simulink model "qref_Model"  (R2024a)
settings: Solver=VariableStepAuto  StartTime=0.0  StopTime=10.0  RelTol=1e-3
libraries: sharedtransform x2, aerolibconvert2 x1
settings Model: Creator=hendr  LastModifiedBy=hendr

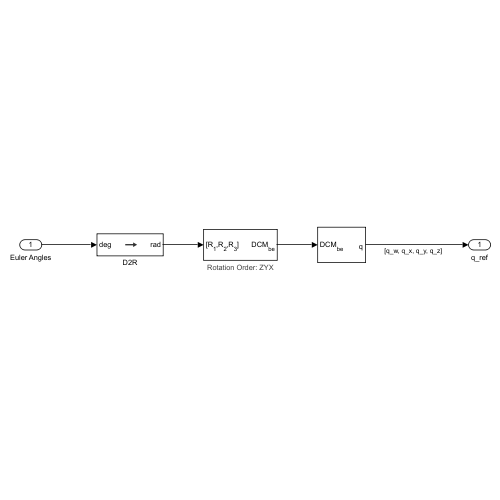
[thumbnail: Simulink's stored preview of the top-level diagram]
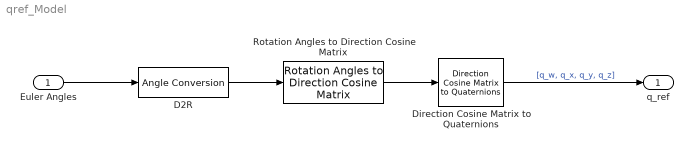
== system qref_Model ==
  Euler Angles : Inport
  D2R : aerolibconvert2/Angle Conversion  IU=deg  OU=rad
  Direction Cosine Matrix to Quaternions : sharedtransform/Direction Cosine Matrix  to Quaternions  aMode=0  action=None  tolerance=eps(2)
      settings: LibrarySourceBlock=|
      | aerolibtransform2/Direction Cosine Matrix
      | to Quaternions
  Rotation Angles to Direction Cosine Matrix : sharedtransform/Rotation Angles to Direction Cosine Matrix  rotationOrder=ZYX  aMode=aMode
  q_ref : Outport
  wires:
  Euler Angles/1 -> D2R/1
  D2R/1 -> Rotation Angles to Direction Cosine Matrix/1
  Rotation Angles to Direction Cosine Matrix/1 -> Direction Cosine Matrix to Quaternions/1
  Direction Cosine Matrix to Quaternions/1 -> q_ref/1  "[q_w, q_x, q_y, q_z]"
